simulink model "batterymodel"  (R2015a)
settings: Solver=ode5  StartTime=0.0  StopTime=PowerInputVector(end,1)  FixedStep=0.2  RelTol=1e-3
values from neighbouring files (symbols this model uses):
  init_SOC = 0.9    [runAndEditMe.m]
  n_cell_parallel = Simulink.Parameter    [runAndEditMe.m]
  n_cell_series = Simulink.Parameter    [runAndEditMe.m]
undefined symbols (not defined in the file or in its folder): bat, becm
settings Model: Creator=rickardarvidsson  LastModifiedBy=rickardarvidsson
settings DataIOCC: LimitDataPoints=off

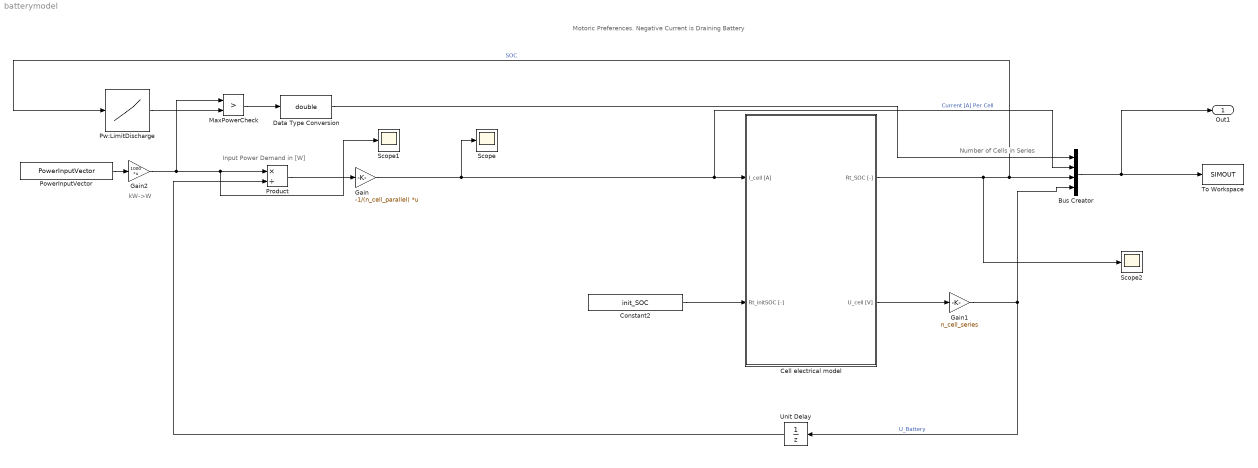
== system batterymodel ==
  note: kW->W
  note: Input Power Demand in [W]
  note: Motoric Preferences. Negative Current is Draining Battery
  note: Number of Cells in Series
  Bus Creator : BusCreator
  Cell electrical model : Subsystem  AncestorBlock=batteryScalable_v1/Cell electrical model
  Constant2 : Constant  Value=init_SOC
  Data Type Conversion : DataTypeConversion  OutDataTypeStr=double
  Gain : Gain  Gain=-1/(n_cell_parallel)  Multiplication=Matrix(K*u)
  Gain1 : Gain  Gain=n_cell_series
  Gain2 : Gain  Gain=1000  Multiplication=Matrix(K*u)
  MaxPowerCheck : RelationalOperator  Operator=>  OutDataTypeStr=boolean
  PowerInputVector : FromWorkspace  VariableName=PowerInputVector
  Product : Product  Inputs=*/  RndMeth=Zero
  Pw:LimitDischarge : Lookup  InputValues=becm.Rt_SOC_x  Table=becm.Pw_limitDischarge_z *1000  LookUpMeth=Interpolation-Use End Values
  Scope : Scope
  Scope1 : Scope
  Scope2 : Scope
      settings: SaveName=ScopeData2
  To Workspace : ToWorkspace  VariableName=SIMOUT  SaveFormat=Structure With Time  SampleTime=-1
  Unit Delay : UnitDelay  InitialCondition=mean(bat.cell.U_OCV_y)*n_cell_series  SampleTime=-1
  Out1 : Outport
  wires:
  Gain/1 -> Scope/1, Bus Creator/2, Cell electrical model/1(I_cell [A])  "Current [A] Per Cell"
  Cell electrical model/2(U_cell [V]) -> Gain1/1
  Gain1/1 -> Bus Creator/4, Unit Delay/1  "U_Battery"
  Constant2/1 -> Cell electrical model/2(Rt_initSOC [-])
  Product/1 -> Gain/1
  Unit Delay/1 -> Product/2
  PowerInputVector/1 -> Gain2/1
  Cell electrical model/1(Rt_SOC [-]) -> Scope2/1, Pw:LimitDischarge/1, Bus Creator/3  "SOC"
  Pw:LimitDischarge/1 -> MaxPowerCheck/2
  Bus Creator/1 -> Out1/1, To Workspace/1
  MaxPowerCheck/1 -> Data Type Conversion/1
  Data Type Conversion/1 -> Bus Creator/1
  Gain2/1 -> MaxPowerCheck/1, Scope1/1, Product/1

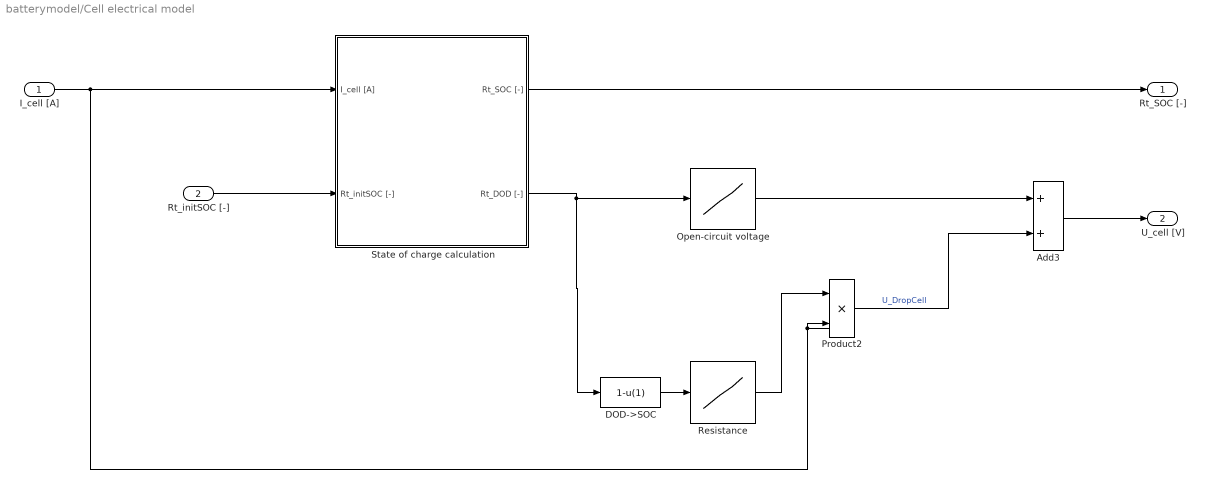
== system batterymodel/Cell electrical model ==
  I_cell [A] : Inport
  Rt_initSOC [-] : Inport  Port=2
  Add3 : Sum
  DOD->SOC : Fcn  Expr=1-u(1)
  Open-circuit voltage : Lookup  InputValues=bat.cell.Rt_DOD_x  Table=bat.cell.U_OCV_y  LookUpMeth=Interpolation-Use End Values
  Product2 : Product  Inputs=**  RndMeth=Zero
  Resistance : Lookup  InputValues=linspace(0,1,7)  Table=bat.cell.R_0_z(:,1)
  State of charge calculation : Subsystem
  Rt_SOC [-] : Outport
  U_cell [V] : Outport  Port=2
  wires:
  State of charge calculation/1(Rt_SOC [-]) -> Rt_SOC [-]/1
  State of charge calculation/2(Rt_DOD [-]) -> Open-circuit voltage/1, DOD->SOC/1
  Open-circuit voltage/1 -> Add3/1
  Add3/1 -> U_cell [V]/1
  Rt_initSOC [-]/1 -> State of charge calculation/2(Rt_initSOC [-])
  Product2/1 -> Add3/2  "U_DropCell"
  DOD->SOC/1 -> Resistance/1
  I_cell [A]/1 -> Product2/2, State of charge calculation/1(I_cell [A])
  Resistance/1 -> Product2/1

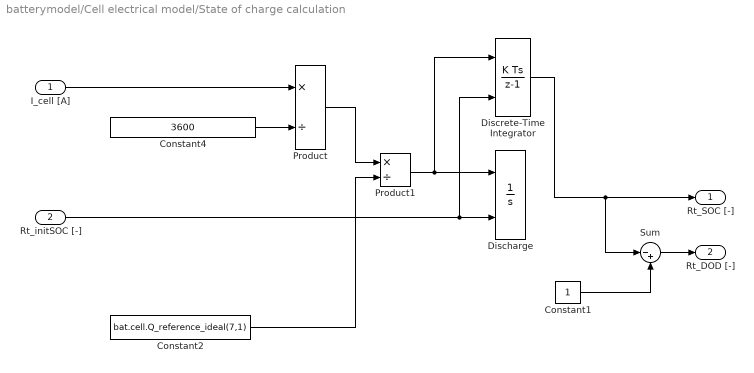
== system batterymodel/Cell electrical model/State of charge calculation ==
  I_cell [A] : Inport
  Rt_initSOC [-] : Inport  Port=2
  Constant1 : Constant
  Constant2 : Constant  Value=bat.cell.Q_reference_ideal(7,1)
  Constant4 : Constant  Value=3600
  Discharge : Integrator  InitialConditionSource=external  InitialCondition=bat.Rt_initialSOC  LimitOutput=on  UpperSaturationLimit=1  LowerSaturationLimit=0
  Discrete-Time Integrator : DiscreteIntegrator  InitialConditionSource=external  InitialConditionSetting=State (most efficient)  SampleTime=0.2
  Product : Product  Inputs=*/  OutMin=-500  OutMax=500  RndMeth=Zero
  Product1 : Product  Inputs=*/  RndMeth=Zero
  Sum : Sum  Inputs=|-+
  Rt_SOC [-] : Outport
  Rt_DOD [-] : Outport  Port=2
  wires:
  I_cell [A]/1 -> Product/1
  Product/1 -> Product1/1
  Constant2/1 -> Product1/2
  Discrete-Time Integrator/1 -> Sum/1, Rt_SOC [-]/1
  Sum/1 -> Rt_DOD [-]/1
  Constant4/1 -> Product/2
  Constant1/1 -> Sum/2
  Rt_initSOC [-]/1 -> Discrete-Time Integrator/2, Discharge/2
  Product1/1 -> Discrete-Time Integrator/1, Discharge/1
